simulink model "PertrubeObserve"  (R2019a)
settings: Solver=VariableStepAuto  StartTime=0.0  StopTime=2.5  RelTol=1e-3
libraries: powerlib x10, powerlib_meascontrol x2, re_lib x1, simulink x1
settings Model: Creator=LOUZAZNI  LastModifiedBy=Blacken

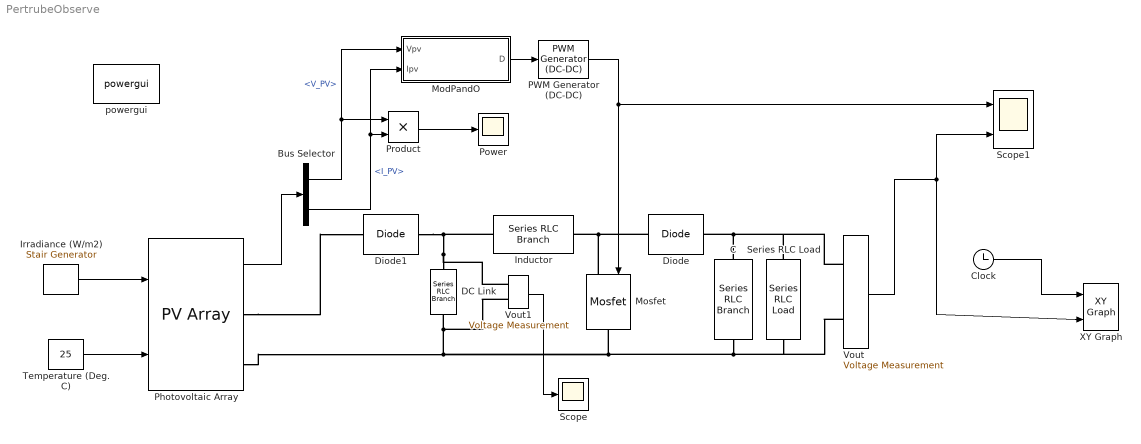
== system PertrubeObserve ==
  Bus Selector : BusSelector  OutputSignals=V_PV,I_PV
  C : powerlib/Elements/Series RLC Branch  LConnTagsString=__new0  RConnTagsString=__new0  BranchType=C  Resistance=1  Inductance=1e-3  SetiL0=off  InitialCurrent=0  Capacitance=50e-6  Setx0=off  InitialVoltage=600  Measurements=None
      settings: SourceProductName=Simscape Electrical
  Clock : Clock
  DC Link : powerlib/Elements/Series RLC Branch  LConnTagsString=__new0  RConnTagsString=__new0  BranchType=C  Resistance=0.001  Inductance=1.0  SetiL0=off  InitialCurrent=0  Capacitance=4000e-6  Setx0=off  InitialVoltage=310  Measurements=None
      settings: SourceProductName=Simscape Electrical
  Diode : powerlib/Power Electronics/Diode  Ron=0.001  Lon=0  Vf=0.8  IC=0  UseSnubber=off  Rs=500  Cs=250e-9  Measurements=off
      settings: SourceProductName=Simscape Electrical
  Diode1 : powerlib/Power Electronics/Diode  Ron=0.001  Lon=0  Vf=0.8  IC=0  UseSnubber=off  Rs=500  Cs=250e-9  Measurements=off
      settings: SourceProductName=Simscape Electrical
  Inductor : powerlib/Elements/Series RLC Branch  LConnTagsString=__new0  RConnTagsString=__new0  BranchType=L  Resistance=0.01  Inductance=4e-4  SetiL0=off  InitialCurrent=5  Capacitance=1e-6  Setx0=off  InitialVoltage=0  Measurements=None
      settings: SourceProductName=Simscape Electrical
  Irradiance (W/m2) : powerlib_meascontrol/Pulse & Signal Generators/Stair Generator  t=[0, 0.5, 1, 1.5, 2]  e=[0.5, 1, 0.8, 0.6, 0.2]*1000  Ts=0.0001
      settings: SourceProductName=Simscape Electrical
  ModPandO : Subsystem
  Mosfet : powerlib/Power Electronics/Mosfet  Ron=0.1  Lon=0  Rd=0.01  Vfd=0  IC=0  Rs=1e5  Cs=inf  Measurements=off
      settings: SourceProductName=Simscape Electrical
  PWM Generator (DC-DC) : powerlib_meascontrol/Pulse & Signal Generators/PWM Generator (DC-DC)  Fsw=10000  Ts=0
      settings: SourceProductName=Simscape Electrical
  Photovoltaic Array : re_lib/Solar/PV Array  Npar=1  Nser=1  PlotType=one module @ 25 deg.C & specified irradiances  S_vec=[800]  Temp_C_vec=[ 50 ]  ModuleName=Kyocera Solar KC200GT  PlotWhenSelected=off  Pm=200.143  Ncell=54  Voc=32.9  Isc=8.21  Vm=26.3  Im=7.61  beta_Voc_pc=-0.35502  alpha_Isc_pc=0.06  beta_Voc=-0.1168  alpha_Isc=0.004926  IL=8.2288  I0=2.3246e-10  nI=0.97736  Rsh=150.6921  Rs=0.34483  BAL=on  Tc=1e-6  Tfilter=5e-5
      settings: SourceProductName=Simscape Electrical
      settings: AttributesFormatString=|
      | %<ModuleName>
      | %<Nser>-module string
      | %<Npar> parallel strings
  Power : Scope
  Product : Product  RndMeth=Zero
  Scope : Scope
  Scope1 : Scope  NumInputPorts=2
  Series RLC Load : powerlib/Elements/Series RLC Load  LConnTagsString=a  RConnTagsString=__new0  NominalVoltage=30  NominalFrequency=50  ActivePower=120  InductivePower=0  CapacitivePower=0  Setx0=off  InitialVoltage=0  SetiL0=off  InitialCurrent=0  Measurements=None  LoadType=constant Z
      settings: SourceProductName=Simscape Electrical
  Temperature (Deg. C) : Constant  Value=25
  Vout : powerlib/Measurements/Voltage Measurement  PhasorSimulation=off  OutputType=Complex  PSBequivalent=0
      settings: SourceProductName=Simscape Electrical
  Vout1 : powerlib/Measurements/Voltage Measurement  PhasorSimulation=off  OutputType=Complex  PSBequivalent=0
      settings: SourceProductName=Simscape Electrical
  XY Graph : simulink/Sinks/XY Graph  xmin=0  xmax=2  ymin=0  ymax=50  st=0.0001
  powergui : powerlib/powergui  Priority=1  SimulationMode=Discrete  SampleTime=5e-7  frequency=60  Iterations=50  frequencyindice=0  Pbase=100e6  ErrMax=1e-4  UnitsV=kV  UnitsW=MW  buscounter=0  FunctionMessages=off  echomessages=off  EnableUseOfTLC=off  CurrentSourceSwitches=off  DisableSnubberDevices=off  DisableRonSwitches=off  DisableVfSwitches=off  DisplayEquations=off  AutomaticDiscreteSolvers=off  SolverType=Tustin/Backward Euler (TBE)  Interpol=off  ExternalGateDelay=off  methode=off  Ts=100  x0status=blocks  SPID=off  SwTol=0  HookPort=off  NonlinearTolerance=0  nMaxIteration=15  ContinueOnMaxIteration=off  RestoreLinks=warning  ResistiveCurrentMeasurement=off  Frange=[0:2:500]  Ylog=off  Xlog=on  ShowGrid=off  save=off  variable=ZData  structure=0  ZoomFFT=off  StartTime=0.0  cycles=1  DisplayStyle=1  fundamental=60  FreqAxis=off  MaxFrequency=1000  frequencyindicesteady=1  RmsSteady=1  display=off
      settings: SourceProductName=Simscape Electrical
  wires:
  Vout1/1 -> Scope/1
  Vout/1 -> XY Graph/2, Scope1/2
  Clock/1 -> XY Graph/1
  Bus Selector/1 -> Product/1, ModPandO/1(Vpv)  "<V_PV>"
  Photovoltaic Array/1 -> Bus Selector/1
  PWM Generator (DC-DC)/1 -> Mosfet/1, Scope1/1
  Bus Selector/2 -> Product/2, ModPandO/2(Ipv)  "<I_PV>"
  Irradiance (W/m2)/1 -> Photovoltaic Array/1
  Temperature (Deg. C)/1 -> Photovoltaic Array/2
  ModPandO/1(D) -> PWM Generator (DC-DC)/1
  Product/1 -> Power/1
  connections:
  Photovoltaic Array/RConn2 -- Vout1/LConn2 -- DC Link/RConn1 -- Mosfet/RConn1 -- Vout/LConn2 -- Series RLC Load/RConn1 -- C/RConn1
  Mosfet/LConn1 -- Inductor/RConn1 -- Diode/LConn1
  Diode1/RConn1 -- Vout1/LConn1 -- DC Link/LConn1 -- Inductor/LConn1
  C/LConn1 -- Diode/RConn1 -- Vout/LConn1 -- Series RLC Load/LConn1
  Photovoltaic Array/RConn1 -- Diode1/LConn1

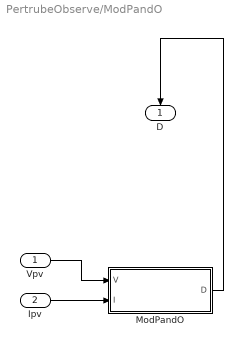
== system PertrubeObserve/ModPandO ==
  Vpv : Inport
  Ipv : Inport  Port=2
  ModPandO : MATLAB Function  TreatAsAtomicUnit=on
  D : Outport
  wires:
  ModPandO/1(D) -> D/1
  Vpv/1 -> ModPandO/1(V)
  Ipv/1 -> ModPandO/2(I)

== matlab function PertrubeObserve/ModPandO/ModPandO ==
  data: D output; V input; I input

% f=1000 hz(G)
function D  = ModPandO(V, I)


Dinit = 0.42;  %Initial value for D output
Dmax = 0.65;   %Maximum value for D
Dmin = 0.1;   %Minimum value for D
deltaD = 0.002; %Increment value used to increase/decrease the duty cycle D

  
persistent Vold Pold Dold M;

dataType = 'double';

if isempty(Vold)
    Vold=0;
    Pold=0;
    Dold=Dinit;
    M=1;
end
P= V*I;
dV= V - Vold;
dP= P - Pold;

M=abs(dP);

if M < 0.005
    D=Dold;
else
    if dP < 0
        if dV < 0
            D = Dold - deltaD*M;
        else
            D = Dold + deltaD*M;
        end
    else
        if dV < 0
            D = Dold + deltaD*M;
        else
            D = Dold - deltaD*M;
        end    
    end

end

if D >= Dmax | D<= Dmin
    D=Dold;
end

Dold=D;
Vold=V;
Pold=P;
